simulink model "exec"  (Simulink 3.00)
libraries: execlib x6
settings Model: MaskType=REX sequence  MaskIconFrame=on  MaskIconOpaque=on  MaskIconRotate=none  MaskIconUnits=autoscale

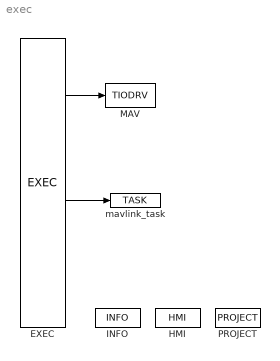
== system exec ==
  EXEC : execlib/EXEC  target=Generic target device  tick=0.001  ntick0=50  ntick1=50  ntick2=100  ntick3=1200  pri0=5  pri1=9  pri2=13  pri3=18  cpu0=-1  cpu1=-1  cpu2=-1  cpu3=-1
  HMI : execlib/HMI  IncludeHMI=on  HmiDir=hmi  SourceDir=hmisrc  GenerateWebWatch=off  GenerateRexHMI=on  RedirectToHMI=on  Compression=on
  INFO : execlib/INFO  Title=MAVLink interface for program.py  Author=UWB
  MAV : execlib/TIODRV  module=MAVLinkDrv  classname=MAVLinkDrv  cfgname=MAVLink.rio  factor=1  stack=10240  pri=3  timer=off  cpu=-1
  PROJECT : execlib/PROJECT  SourcesOnTarget=off  TargetURL=147.228.113.63  LibraryPath=../library
  mavlink_task : execlib/TASK  factor=1  start=0  stop=1  stack=10240  MDLOPEN=on
  wires:
  EXEC/2 -> MAV/1
  EXEC/5 -> mavlink_task/1
